simulink model "rmspec"  (Simulink 7.0)
settings: Solver=ode45  StartTime=0.0  StopTime=200  RelTol=1e-3
undefined symbols (not defined in the file): pfb_coeff_gen_calc
libraries: xbsIndex_r4 x3092, casper_library x230, xps_library x24
(part 1 of 33)
settings Model: Creator=dave  LastModifiedBy=dave

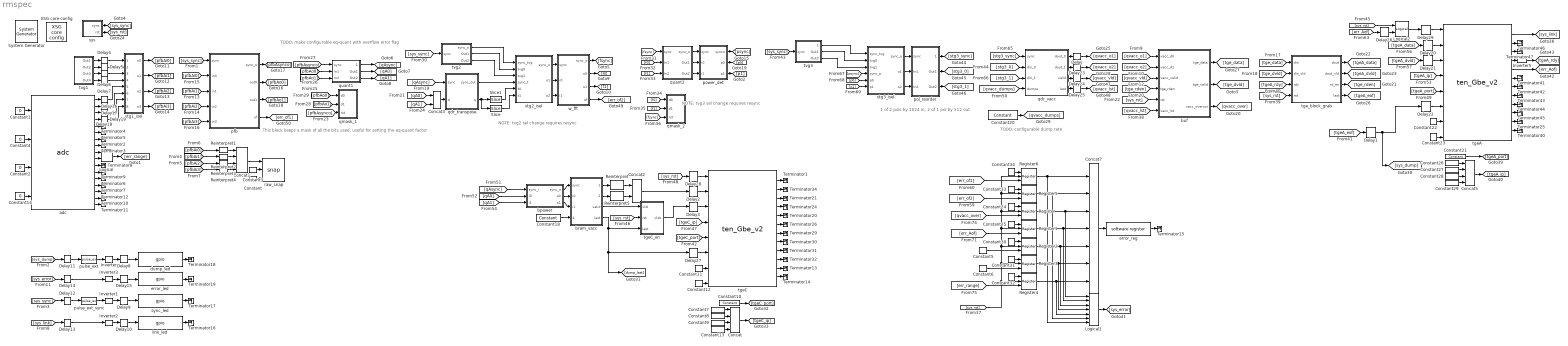
== system rmspec ==
  note: TODO: make configurable eq-quant with
      | overflow error flag
  note: This block keeps a mask of all the bits used,
      | useful for setting the eq-quant factor
  note: NOTE: tvg2 sel change
      | requires resync
  note: 1 of 2 pols by 1024 in,
      | 2 of 1 pol by 512 out
  note: NOTE: tvg3 sel change
      | requires resync
  note: TODO: configurable dump rate
  " System Generator" : xbsIndex_r4/ System Generator  Tag=genX  SystemSampleTime=-1  xilinxfamily=virtex5  part=xc5vsx95t  speed=-1  package=ff1136  synthesis_tool=XST  clock_wrapper=Clock Enables  directory=./rmspec/sysgen  testbench=off  simulink_period=1  sysclk_period=5  dcm_input_clock_period=100  incr_netlist=off  trim_vbits=Everywhere in SubSystem  dbl_ovrd=According to Block Masks  core_generation=According to Block Masks  run_coregen=off  deprecated_control=off  eval_field=0  block_type=sysgen
      settings: block_version=10.1.3
  Concat : xbsIndex_r4/Concat  num_inputs=4  dbl_ovrd=off  block_type=concat
      settings: block_version=10.1.3
  Concat1 : xbsIndex_r4/Concat  num_inputs=4  dbl_ovrd=off  block_type=concat
      settings: block_version=10.1.3
  Concat2 : xbsIndex_r4/Concat  num_inputs=2  dbl_ovrd=off  block_type=concat
      settings: block_version=10.1.3
  Concat3 : xbsIndex_r4/Concat  num_inputs=2  dbl_ovrd=off  block_type=concat
      settings: block_version=10.1.3
  Concat5 : xbsIndex_r4/Concat  num_inputs=4  dbl_ovrd=off  block_type=concat
      settings: block_version=10.1.3
  Concat7 : xbsIndex_r4/Concat  num_inputs=7  dbl_ovrd=off  block_type=concat
      settings: block_version=10.1.3
  Constant : xbsIndex_r4/Constant  arith_type=Boolean  const=1  n_bits=16  bin_pt=14  explicit_period=on  period=1  equ=P=C  opselect=C  inp2=PCIN>>17  opr=+  inp1=P  carry=CIN  dbl_ovrd=off  block_type=constant
  Constant{1..2,4,14} (4 alike) : Constant  Value=0  OutDataType=sfix(16)  OutScaling=2^0
  Constant10 : xbsIndex_r4/Constant  arith_type=Unsigned  const=10002  n_bits=16  bin_pt=0  explicit_period=off  period=1  equ=P=C  opselect=C  inp2=PCIN>>17  opr=+  inp1=P  carry=CIN  dbl_ovrd=off  block_type=constant
  Constant{11..12,22..25,30..34} (11 alike) : xbsIndex_r4/Constant  arith_type=Boolean  const=1  n_bits=16  bin_pt=14  explicit_period=off  period=1  equ=P=C  opselect=C  inp2=PCIN>>17  opr=+  inp1=P  carry=CIN  dbl_ovrd=off  block_type=constant
  Constant13 : xbsIndex_r4/Constant  arith_type=Unsigned  const=2  n_bits=8  bin_pt=0  explicit_period=off  period=1  equ=P=C  opselect=C  inp2=PCIN>>17  opr=+  inp1=P  carry=CIN  dbl_ovrd=off  block_type=constant
  Constant18 : xbsIndex_r4/Constant  arith_type=Unsigned  const=2^23 - 2  n_bits=32  bin_pt=0  explicit_period=off  period=1  equ=P=C  opselect=C  inp2=PCIN>>17  opr=+  inp1=P  carry=CIN  dbl_ovrd=off  block_type=constant
  Constant20 : xbsIndex_r4/Constant  arith_type=Unsigned  const=(2^10)*(2^(10-1))*(2^9) - 2  n_bits=32  bin_pt=0  explicit_period=on  period=1  equ=P=C  opselect=C  inp2=PCIN>>17  opr=+  inp1=P  carry=CIN  dbl_ovrd=off  block_type=constant
  Constant21 : xbsIndex_r4/Constant  arith_type=Unsigned  const=10000  n_bits=16  bin_pt=0  explicit_period=off  period=1  equ=P=C  opselect=C  inp2=PCIN>>17  opr=+  inp1=P  carry=CIN  dbl_ovrd=off  block_type=constant
  Constant26 : xbsIndex_r4/Constant  arith_type=Unsigned  const=192  n_bits=8  bin_pt=0  explicit_period=off  period=1  equ=P=C  opselect=C  inp2=PCIN>>17  opr=+  inp1=P  carry=CIN  dbl_ovrd=off  block_type=constant
  Constant27 : xbsIndex_r4/Constant  arith_type=Unsigned  const=168  n_bits=8  bin_pt=0  explicit_period=off  period=1  equ=P=C  opselect=C  inp2=PCIN>>17  opr=+  inp1=P  carry=CIN  dbl_ovrd=off  block_type=constant
  Constant28 : xbsIndex_r4/Constant  arith_type=Unsigned  const=5  n_bits=8  bin_pt=0  explicit_period=off  period=1  equ=P=C  opselect=C  inp2=PCIN>>17  opr=+  inp1=P  carry=CIN  dbl_ovrd=off  block_type=constant
  Constant29 : xbsIndex_r4/Constant  arith_type=Unsigned  const=2  n_bits=8  bin_pt=0  explicit_period=off  period=1  equ=P=C  opselect=C  inp2=PCIN>>17  opr=+  inp1=P  carry=CIN  dbl_ovrd=off  block_type=constant
  Constant3 : xbsIndex_r4/Constant  arith_type=Boolean  const=0  n_bits=16  bin_pt=14  explicit_period=on  period=1  equ=P=C  opselect=C  inp2=PCIN>>17  opr=+  inp1=P  carry=CIN  dbl_ovrd=off  block_type=constant
  Constant5 : xbsIndex_r4/Constant  arith_type=Boolean  const=0  n_bits=16  bin_pt=14  explicit_period=on  period=1  equ=P=C  opselect=C  inp2=PCIN>>17  opr=+  inp1=P  carry=CIN  dbl_ovrd=off  block_type=constant
  Constant6 : xbsIndex_r4/Constant  arith_type=Boolean  const=0  n_bits=16  bin_pt=14  explicit_period=on  period=1  equ=P=C  opselect=C  inp2=PCIN>>17  opr=+  inp1=P  carry=CIN  dbl_ovrd=off  block_type=constant
  Constant7 : xbsIndex_r4/Constant  arith_type=Unsigned  const=192  n_bits=8  bin_pt=0  explicit_period=off  period=1  equ=P=C  opselect=C  inp2=PCIN>>17  opr=+  inp1=P  carry=CIN  dbl_ovrd=off  block_type=constant
  Constant8 : xbsIndex_r4/Constant  arith_type=Unsigned  const=168  n_bits=8  bin_pt=0  explicit_period=off  period=1  equ=P=C  opselect=C  inp2=PCIN>>17  opr=+  inp1=P  carry=CIN  dbl_ovrd=off  block_type=constant
  Constant9 : xbsIndex_r4/Constant  arith_type=Unsigned  const=5  n_bits=8  bin_pt=0  explicit_period=off  period=1  equ=P=C  opselect=C  inp2=PCIN>>17  opr=+  inp1=P  carry=CIN  dbl_ovrd=off  block_type=constant
  Delay{,1,4..19,22..26} (23 alike) : xbsIndex_r4/Delay  en=off  latency=1  dbl_ovrd=off  reg_retiming=off  block_type=delay
  Delay{2..3,20..21,27..29} (7 alike) : xbsIndex_r4/Delay  en=off  latency=2  dbl_ovrd=off  reg_retiming=off  block_type=delay
  Inverter{,1..3,5} (5 alike) : xbsIndex_r4/Inverter  en=off  latency=0  dbl_ovrd=off  block_type=inv
  Logical : xbsIndex_r4/Logical  logical_function=OR  inputs=2  en=off  latency=0  precision=Full  arith_type=Unsigned  n_bits=16  bin_pt=0  align_bp=on  dbl_ovrd=off  block_type=logical
  Logical1 : xbsIndex_r4/Logical  logical_function=OR  inputs=7  en=off  latency=1  precision=Full  arith_type=Unsigned  n_bits=16  bin_pt=0  align_bp=on  dbl_ovrd=off  block_type=logical
  Logical2 : xbsIndex_r4/Logical  logical_function=OR  inputs=2  en=off  latency=0  precision=Full  arith_type=Unsigned  n_bits=16  bin_pt=0  align_bp=on  dbl_ovrd=off  block_type=logical
  Register{,1..6} (7 alike) : xbsIndex_r4/Register  init=0  rst=on  en=on  dbl_ovrd=off  block_type=register
  Reinterpret{,1..5} (6 alike) : xbsIndex_r4/Reinterpret  force_arith_type=on  arith_type=Unsigned  force_bin_pt=on  bin_pt=0  block_type=reinterpret
      settings: infoedit="Changes signal type without altering the binary representation.   You can changed the signal between signed and unsigned, and relocate the binary point.<P><P>Hardware notes: In hardware this block costs nothing.<P><P>Example:  Suppose the input is 6 bits wide, signed, with 2 fractional bits, and the output is forced to unsigned with 0 fractional bits.  Then an input of -2.0 (1110.00 in binary 2's complement) becomes an output of 56 (111000 in binary)."  block_version=10.1.3
  Slice : xbsIndex_r4/Slice  nbits=18  boolean_output=off  mode=Lower Bit Location + Width  bit1=0  base1=LSB of Input  bit0=0  base0=LSB of Input  dbl_ovrd=off  block_type=slice
      settings: infoedit="Extracts a given range of bits from each input sample and presents it at the output.  The output type is ordinarily unsigned with binary point at zero, but can be Boolean when the slice is one bit wide.<P><P>Hardware notes: In hardware this block costs nothing."  block_version=10.1.3
  Slice1 : xbsIndex_r4/Slice  nbits=18  boolean_output=off  mode=Lower Bit Location + Width  bit1=0  base1=LSB of Input  bit0=18  base0=LSB of Input  dbl_ovrd=off  block_type=slice
      settings: infoedit="Extracts a given range of bits from each input sample and presents it at the output.  The output type is ordinarily unsigned with binary point at zero, but can be Boolean when the slice is one bit wide.<P><P>Hardware notes: In hardware this block costs nothing."  block_version=10.1.3
  Terminator{1..21,24..26,29..32,34,40..47} (37 alike) : Terminator
  XSG core config : xps_library/XSG core config  Tag=xps:xsg  SystemSampleTime=-1  hw_sys=ROACH:sx95t  ibob_linux=off  clk_src=adc0_clk  iBOB_clk_src=sys_clk  BEE2_ctrl_clk_src=sys_clk  BEE2_usr_clk_src=sys_clk  ROACH_clk_src=adc0_clk  CORR_clk_src=sys_clk  gpio_clk_io_group=iBOB:sma  gpio_clk_bit_index=0  clk_rate=200  sample_period=1  synthesis_tool=XST  mpc_type=powerpc440_ext
  adc : xps_library/adc  Tag=xps:adc  SystemSampleTime=-1  adc_brd=adc0  adc_clk_rate=800  adc_interleave=off  sample_period=1
  bpower : Subsystem  mask{bits=9}
  bram_vacc : Subsystem  mask{n_chans=512}
      mask prompts: n_chans "Number of Channels"
  buf : Subsystem  mask{fftsize=10, nochan=10}
      mask prompts: fftsize "fftsize (2^n)"; nochan "nochan (2^n)"
  dump_led : xps_library/gpio  Tag=xps:gpio  SystemSampleTime=-1  io_group=ROACH:led  io_dir=out  arith_type=Boolean  bitwidth=1  bin_pt=0  bit_index=0  sample_period=1  use_single_ended=off  use_ddr=off  reg_iob=on  reg_clk_phase=0  termination=None
      link override convert: arith_type=Boolean  n_bits=1  bin_pt=0
  error_led : xps_library/gpio  Tag=xps:gpio  SystemSampleTime=-1  io_group=ROACH:led  io_dir=out  arith_type=Boolean  bitwidth=1  bin_pt=0  bit_index=1  sample_period=1  use_single_ended=off  use_ddr=off  reg_iob=on  reg_clk_phase=0  termination=None
      link override convert: arith_type=Boolean  n_bits=1  bin_pt=0
  error_reg : xps_library/software register  Tag=xps:sw_reg  SystemSampleTime=-1  io_dir=To Processor  arith_type=Unsigned  bitwidth=32  bin_pt=0  sample_period=1  gw_name=rmspec_error_reg_user_data_in
      link override convert: arith_type=Unsigned  n_bits=32  bin_pt=0
  link_led : xps_library/gpio  Tag=xps:gpio  SystemSampleTime=-1  io_group=ROACH:led  io_dir=out  arith_type=Boolean  bitwidth=1  bin_pt=0  bit_index=3  sample_period=1  use_single_ended=off  use_ddr=off  reg_iob=on  reg_clk_phase=0  termination=None
      link override convert: arith_type=Boolean  n_bits=1  bin_pt=0
  pfb : Subsystem
  pol_reorder : Subsystem
  power_det : Subsystem
  pulse_ext : casper_library/Misc/pulse_ext  SystemSampleTime=-1  pulse_len=2^25
  pulse_ext_sync : casper_library/Misc/pulse_ext  SystemSampleTime=-1  pulse_len=2^20
  qdr_transpose : Subsystem  AncestorBlock=casper_library/Reorder/qdr_transpose  mask{idepth=9, odepth=10, which_qdr=qdr0}
      link override reorder: map=[0 1 2 3]  n_inputs=2
      mask prompts: idepth "Input blocksize (2^n)"; odepth "Output blocksize (2^n)"; which_qdr "QDR Chip"
      mask init:
      | new_map = tostring([[0:2^odepth-1]*2 [0:2^odepth-1]*2 + 1]);
      | set_param([gcb, '/reorder'], 'map', new_map);
      | set_param([gcb, '/qdr'], 'which_qdr', which_qdr);
      mask StyleString: edit,edit,popup(qdr0|qdr1)
  qdr_vacc : Subsystem  mask{n_chans=(2^10)*(2^(10-1)), which_qdr=1, add_lat=3}
      mask prompts: n_chans "Vector Length"; which_qdr "QDR Chip"; add_lat "add_latency"
      mask init:
      | set_param([gcb, '/qdr_delay'], 'which_qdr', sprintf('%d',which_qdr));
  qmask_1 : Subsystem
  qmask_2 : Subsystem
  quant1 : Subsystem  mask{fact=0, bits=9}
      mask prompts: fact "fact (2^n)"; bits "quant bits"
  quant2 : Subsystem  mask{fact=0, bits=18}
      mask prompts: fact "fact (2^n)"; bits "quant bits"
  raw_snap : casper_library/Scopes/snap  SystemSampleTime=-1  nsamples=11
      link override addr/convert: arith_type=Unsigned  n_bits=32  bin_pt=0
      link override bram/convert_din: arith_type=Unsigned
      link override bram/mem/sim_data_in: arith_type=Unsigned
      link override bram/pfb1_tv_raw_snap_bram_data_out: arith_type=Unsigned
      link override bram/rmspec_raw_snap_bram_data_out: arith_type=Unsigned
      link override bram/roach_mspec_raw_snap_bram_data_out: arith_type=Unsigned
      link override bram/stg1_raw_snap_bram_data_out: arith_type=Unsigned
      link override ctrl/pfb1_tv_raw_snap_ctrl_user_data_out: arith_type=Unsigned  n_bits=32  bin_pt=0  period=1
      link override ctrl/rmspec_raw_snap_ctrl_user_data_out: arith_type=Unsigned  n_bits=32  bin_pt=0  period=1
      link override ctrl/roach_mspec_raw_snap_ctrl_user_data_out: arith_type=Unsigned  n_bits=32  bin_pt=0  period=1
      link override ctrl/stg1_raw_snap_ctrl_user_data_out: arith_type=Unsigned  n_bits=32  bin_pt=0  period=1
  stg1_isel : Subsystem
  stg2_isel : Subsystem
  stg3_isel : Subsystem
  sync_led : xps_library/gpio  Tag=xps:gpio  SystemSampleTime=-1  io_group=ROACH:led  io_dir=out  arith_type=Boolean  bitwidth=1  bin_pt=0  bit_index=2  sample_period=1  use_single_ended=off  use_ddr=off  reg_iob=on  reg_clk_phase=0  termination=None
      link override convert: arith_type=Boolean  n_bits=1  bin_pt=0
  sys : Subsystem
  tgeA : xps_library/ten_Gbe_v2  Tag=xps:tengbe_v2  SystemSampleTime=-1  port=0  rx_dist_ram=on  show_param=on  pre_emph=3  swing=800  fab_en=on  fab_mac=hex2dec('123456780000')  fab_ip=192*(2^24) + 168*(2^16) + 5*(2^8) + 20*(2^0)  fab_udp=10000  fab_gate=1  cpu_rx_en=off  cpu_tx_en=off
  tgeC : xps_library/ten_Gbe_v2  Tag=xps:tengbe_v2  SystemSampleTime=-1  port=2  rx_dist_ram=on  show_param=on  pre_emph=3  swing=800  fab_en=on  fab_mac=hex2dec('123456780002')  fab_ip=192*(2^24) + 168*(2^16) + 5*(2^8) + 20*(2^0)  fab_udp=10002  fab_gate=1  cpu_rx_en=off  cpu_tx_en=off
  tgeC_en : Subsystem
  tge_block_grab : Subsystem
  tvg1 : Subsystem  mask{lev=0.1}
  tvg2 : Subsystem
  tvg3 : Subsystem  mask{fftsize=10, nochan=10, vaccwidth=18, dumps=9}
      mask prompts: fftsize "fftsize (2^n)"; nochan "nochan (2^n)"; dumps "dumps (2^n)"
  w_fft : Subsystem
  wires:
  [pfbAi0] -> Reinterpret1/1
  [pfbAi1] -> Reinterpret2/1
  [pfbAi2] -> Reinterpret3/1
  [pfbAi3] -> Reinterpret4/1
  Concat1/1 -> raw_snap/1
  Constant/1 -> raw_snap/3
  Constant3/1 -> raw_snap/2
  Reinterpret1/1 -> Concat1/1
  Reinterpret2/1 -> Concat1/2
  Reinterpret3/1 -> Concat1/3
  Reinterpret4/1 -> Concat1/4
  [pfbAo0] -> quant1/2(In1)
  [pfbAo1] -> quant1/3(In2)
  [pfbAsynco] -> quant1/1(sync)
  [pfbAi0] -> pfb/2(in0)
  [pfbAi1] -> pfb/3(in1)
  [pfbAi2] -> pfb/4(in2)
  [pfbAi3] -> pfb/5(in3)
  pfb/1(sync_o) -> [pfbAsynco]
  pfb/2(out0) -> [pfbAo0]
  pfb/3(out1) -> [pfbAo1]
  [sys_sync] -> pfb/1(sync)
  pulse_ext/1 -> Inverter/1
  [sys_dump] -> Delay11/1
  [sys_sync] -> Delay12/1
  [sys_link] -> Delay13/1
  tvg1/1(Out1) -> Delay4/1
  tvg1/2(Out2) -> Delay5/1
  tvg1/3(Out3) -> Delay6/1
  tvg1/4(Out4) -> Delay7/1
  pfb/4(of) -> [err_of1]
  Delay8/1 -> dump_led/1
  Delay9/1 -> sync_led/1
  Delay10/1 -> link_led/1
  Delay11/1 -> pulse_ext/1
  Delay12/1 -> pulse_ext_sync/1
  Delay13/1 -> Inverter2/1
  Inverter/1 -> Delay8/1
  Inverter1/1 -> Delay9/1
  Inverter2/1 -> Delay10/1
  quant1/1(sync_o) -> [qAsync]
  quant1/2(Out1) -> [qA0]
  quant1/3(Out2) -> [qA1]
  Constant1/1 -> adc/1
  Constant2/1 -> adc/3
  Constant4/1 -> adc/2
  Constant14/1 -> adc/4
  adc/1 -> Delay16/1
  adc/2 -> Delay17/1
  adc/3 -> Delay18/1
  adc/4 -> Delay19/1
  adc/5 -> Terminator4/1
  adc/6 -> Terminator5/1
  adc/7 -> Terminator2/1
  adc/8 -> Terminator3/1
  sys/1(sync) -> [sys_sync]
  sys/2(rst) -> [sys_rst]
  adc/9 -> Logical/1
  adc/10 -> Logical/2
  stg1_isel/1(o0) -> [pfbAi0]
  stg1_isel/2(o1) -> [pfbAi1]
  stg1_isel/3(o2) -> [pfbAi2]
  stg1_isel/4(o3) -> [pfbAi3]
  Logical/1 -> [err_range]
  adc/11 -> Terminator8/1
  adc/12 -> Terminator9/1
  adc/13 -> Terminator6/1
  adc/14 -> Terminator7/1
  adc/15 -> Terminator12/1
  adc/16 -> Terminator10/1
  adc/17 -> Terminator11/1
  Delay16/1 -> stg1_isel/5(adc0)
  Delay17/1 -> stg1_isel/6(adc1)
  Delay18/1 -> stg1_isel/7(adc2)
  Delay19/1 -> stg1_isel/8(adc3)
  dump_led/1 -> Terminator18/1
  sync_led/1 -> Terminator17/1
  link_led/1 -> Terminator16/1
  [sys_error] -> Delay14/1
  Delay15/1 -> error_led/1
  Delay14/1 -> Inverter3/1
  Inverter3/1 -> Delay15/1
  error_led/1 -> Terminator19/1
  [pfbAo0] -> qmask_1/1(d0)
  [pfbAo1] -> qmask_1/2(d1)
  [pfbAsynco] -> qmask_1/3(rst)
  Delay4/1 -> stg1_isel/1(tvg0)
  Delay5/1 -> stg1_isel/2(tvg1)
  Delay6/1 -> stg1_isel/3(tvg2)
  Delay7/1 -> stg1_isel/4(tvg3)
  pulse_ext_sync/1 -> Inverter1/1
  [qA0] -> Concat3/1
  [qA1] -> Concat3/2
  [qAsync] -> qdr_transpose/1(sync)
  Concat3/1 -> qdr_transpose/2(d)
  qdr_transpose/2(q) -> Slice1/1, Slice/1
  [sys_sync] -> tvg2/1(sync)
  tvg2/1(sync_o) -> stg2_isel/1(sync_tvg)
  tvg2/2(Out1) -> stg2_isel/2(tvg0)
  tvg2/3(Out2) -> stg2_isel/3(tvg1)
  qdr_transpose/1(sync_out) -> stg2_isel/4(sync_t)
  Slice1/1 -> stg2_isel/5(t0)
  Slice/1 -> stg2_isel/6(t1)
  stg2_isel/1(sync_o) -> w_fft/1(sync)
  stg2_isel/2(o1) -> w_fft/2(i0)
  stg2_isel/3(o2) -> w_fft/3(i1)
  w_fft/1(sync_o) -> [fsync]
  w_fft/2(o0) -> [f0]
  w_fft/3(o1) -> [f1]
  [fsync] -> quant2/1(sync)
  [f0] -> quant2/2(In1)
  [f1] -> quant2/3(In2)
  [f0] -> qmask_2/1(d0)
  [f1] -> qmask_2/2(d1)
  [fsync] -> qmask_2/3(rst)
  power_det/1(synco) -> [psync]
  power_det/2(p0) -> [p0]
  power_det/3(p1) -> [p1]
  [qvacc_dumps] -> qdr_vacc/4(dumps)
  [sys_sync] -> tvg3/1(sync)
  tgeA/1 -> [sys_link]
  tgeA/2 -> Terminator46/1
  [tgeA_ip] -> tgeA/4
  [tgeA_port] -> tgeA/5
  Constant26/1 -> Concat5/1
  Constant27/1 -> Concat5/2
  Constant28/1 -> Concat5/3
  Constant29/1 -> Concat5/4
  Concat5/1 -> [tgeA_ip]
  Constant21/1 -> [tgeA_port]
  tgeA/4 -> Inverter5/1
  tgeA/6 -> Terminator41/1
  tgeA/7 -> Terminator42/1
  tgeA/8 -> Terminator43/1
  tgeA/9 -> Terminator44/1
  tgeA/10 -> Terminator45/1
  tgeA/11 -> Terminator25/1
  tgeA/12 -> Terminator40/1
  Constant22/1 -> tgeA/7
  Constant23/1 -> tgeA/8
  Delay20/1 -> tgeA/2
  Delay21/1 -> tgeA/3
  Delay22/1 -> tgeA/6
  tgeA/5 -> [err_Aof]
  [err_Aof] -> Delay26/1
  Inverter5/1 -> [tgeA_rdy]
  [stg3_sync] -> qdr_vacc/1(sync)
  [stg3_0] -> qdr_vacc/2(din_0)
  [stg3_1] -> qdr_vacc/3(din_1)
  qdr_vacc/1(dout_0) -> Delay/1
  qdr_vacc/2(dout_1) -> Delay23/1
  qdr_vacc/3(valid) -> Delay24/1
  Constant20/1 -> [qvacc_dumps]
  [tgeA_data] -> Delay20/1
  [tgeA_dvld] -> Delay21/1
  Constant24/1 -> Register/1
  Constant25/1 -> Register1/1
  Register/1 -> Concat7/3, Logical1/1
  Register1/1 -> Concat7/4, Logical1/2
  Logical1/1 -> [sys_error]
  error_reg/1 -> Terminator15/1
  Delay/1 -> [qvacc_o1]
  Delay23/1 -> [qvacc_o2]
  pol_reorder/1(sync_o) -> [stg3_sync]
  pol_reorder/2(Out1) -> [stg3_0]
  pol_reorder/3(Out2) -> [stg3_1]
  Delay24/1 -> [qvacc_vld]
  Delay25/1 -> [qvacc_lst]
  qdr_vacc/4(last) -> Delay25/1
  [sys_rst] -> Logical2/1
  Delay26/1 -> Logical2/2
  Logical2/1 -> Delay29/1
  [psync] -> stg3_isel/4(sync_p)
  [p0] -> stg3_isel/5(p0)
  tvg3/1(sync_o) -> stg3_isel/1(sync_tvg)
  tvg3/2(Out1) -> stg3_isel/2(tvg0)
  tvg3/3(Out2) -> stg3_isel/3(tvg1)
  [p1] -> stg3_isel/6(p1)
  stg3_isel/1(sync_o) -> pol_reorder/1(sync)
  stg3_isel/2(o1) -> pol_reorder/2(In1)
  stg3_isel/3(o2) -> pol_reorder/3(In2)
  tgeA/3 -> Terminator47/1
  Constant30/1 -> Register2/1
  Constant31/1 -> Register3/1
  Register2/1 -> Concat7/5, Logical1/3
  Register3/1 -> Concat7/6, Logical1/4
  Constant32/1 -> Register4/1
  Register4/1 -> Concat7/7, Logical1/5
  Delay29/1 -> tgeA/1
  w_fft/4(of) -> [err_of2]
  Constant33/1 -> Register5/1
  Constant34/1 -> Register6/1
  Concat7/1 -> error_reg/1
  Register6/1 -> Concat7/1, Logical1/7
  Register5/1 -> Concat7/2, Logical1/6
  [sys_rst] -> Register6/2, Register5/2, Register/2, Register1/2, Register2/2, Register3/2, Register4/2
  [err_of1] -> Register6/3
  [err_of2] -> Register5/3
  [qvacc_over] -> Register/3
  [err_Aof] -> Register1/3
  Constant6/1 -> Register3/3
  [err_range] -> Register4/3
  Constant5/1 -> Register2/3
  [tgeA_rdy] -> tge_block_grab/3(rdy)
  buf/1(tge_data) -> [tge_data]
  buf/2(tge_valid) -> [tge_dvld]
  buf/3(vacc_overrun) -> [qvacc_over]
  [tge_data] -> tge_block_grab/1(din)
  [tge_dvld] -> tge_block_grab/2(din_vld)
  tge_block_grab/3(rd_en) -> [tge_rden]
  tge_block_grab/1(dout) -> [tgeA_data]
  tge_block_grab/2(dout_vld) -> [tgeA_dvld]
  tge_block_grab/4(last) -> [tgeA_eof]
  [qvacc_o1] -> buf/1(vacc_d0)
  [qvacc_o2] -> buf/2(vacc_d1)
  [qvacc_vld] -> buf/3(vacc_valid)
  [tge_rden] -> buf/4(tge_rden)
  [sys_rst] -> buf/5(rst)
  [qvacc_lst] -> buf/6(vacc_lst)
  [sys_rst] -> tge_block_grab/4(rst)
  [tgeA_eof] -> Delay1/1
  Delay1/1 -> Delay22/1, [sys_dump]
  Constant18/1 -> bram_vacc/4(dumps)
  tgeC/1 -> Terminator1/1
  tgeC/2 -> Terminator34/1
  tgeC/3 -> Terminator21/1
  [tgeC_ip] -> tgeC/4
  [tgeC_port] -> tgeC/5
  Constant7/1 -> Concat/1
  Constant8/1 -> Concat/2
  Constant9/1 -> Concat/3
  Constant13/1 -> Concat/4
  Concat/1 -> [tgeC_ip]
  Constant10/1 -> [tgeC_port]
  tgeC/4 -> Terminator24/1
  tgeC/6 -> Terminator26/1
  tgeC/7 -> Terminator29/1
  tgeC/8 -> Terminator30/1
  tgeC/9 -> Terminator31/1
  tgeC/10 -> Terminator32/1
  tgeC/11 -> Terminator13/1
  tgeC/12 -> Terminator14/1
  Constant11/1 -> tgeC/7
  Constant12/1 -> tgeC/8
  Delay2/1 -> tgeC/2
  Delay3/1 -> tgeC/3
  Delay27/1 -> tgeC/6
  tgeC/5 -> Terminator20/1
  bpower/1(sync_o) -> bram_vacc/1(sync)
  bpower/2(o0) -> bram_vacc/2(i0)
  bpower/3(o1) -> bram_vacc/3(i1)
  [sys_rst] -> Delay28/1
  bram_vacc/1(dout_0) -> Reinterpret/1
  bram_vacc/2(dout_1) -> Reinterpret5/1
  [sys_rst] -> tgeC_en/2(rst)
  bram_vacc/3(valid) -> tgeC_en/1(vldi)
  bram_vacc/4(last) -> tgeC_en/3(last), Delay27/1, [dump_last]
  Concat2/1 -> Delay2/1
  tgeC_en/1(vldo) -> Delay3/1
  Reinterpret/1 -> Concat2/1
  Reinterpret5/1 -> Concat2/2
  Delay28/1 -> tgeC/1
  [qAsync] -> bpower/1(sync_i)
  [qA0] -> bpower/2(i0)
  [qA1] -> bpower/3(i1)
  quant2/1(sync_o) -> power_det/1(sync)
  quant2/2(Out1) -> power_det/2(i0)
  quant2/3(Out2) -> power_det/3(i1)

== system rmspec/bpower ==
  sync_i : Inport
  i0 : Inport  Port=2
  i1 : Inport  Port=3
  Delay : xbsIndex_r4/Delay  en=off  latency=3  dbl_ovrd=off  reg_retiming=off  block_type=delay
  Scope : Scope  NumInputPorts=3
      settings: YMin=-5~-5~-5  YMax=5~5~5
  power0 : casper_library/Misc/power  SystemSampleTime=-1  BitWidth=bits  add_latency=1  mult_latency=2
  power1 : casper_library/Misc/power  SystemSampleTime=-1  BitWidth=bits  add_latency=1  mult_latency=2
      link override power_adder: mode=Addition  use_carryin=off  use_carryout=off  en=off  latency=add_latency  precision=User Defined  arith_type=Unsigned  n_bits=BitWidth * 2  bin_pt=BitWidth * 2 - 1  quantization=Truncate  overflow=Saturate  dbl_ovrd=off  use_behavioral_HDL=on  pipelined=off  use_rpm=on  hw_selection=Fabric
      link override power_adder: xl_area=[0, 0, 0, 0, 0, 0, 0]
  sync_o : Outport
  o0 : Outport  Port=2
  o1 : Outport  Port=3
  wires:
  sync_i/1 -> Delay/1
  Delay/1 -> sync_o/1, Scope/1
  i0/1 -> power0/1
  i1/1 -> power1/1
  power0/1 -> o0/1, Scope/2
  power1/1 -> o1/1, Scope/3

== system rmspec/bram_vacc ==
  sync : Inport
  i0 : Inport  Port=2
  i1 : Inport  Port=3
  dumps : Inport  Port=4
  Constant2 : xbsIndex_r4/Constant  arith_type=Unsigned  const=0  n_bits=32  bin_pt=0  explicit_period=on  period=1  equ=P=C  opselect=C  inp2=PCIN>>17  opr=+  inp1=P  carry=CIN  dbl_ovrd=off  block_type=constant
  Delay1 : xbsIndex_r4/Delay  en=off  latency=1  dbl_ovrd=off  reg_retiming=off  block_type=delay
  Delay2 : xbsIndex_r4/Delay  en=off  latency=1  dbl_ovrd=off  reg_retiming=off  block_type=delay
  Logical : xbsIndex_r4/Logical  logical_function=OR  inputs=2  en=off  latency=0  precision=Full  arith_type=Unsigned  n_bits=16  bin_pt=0  align_bp=on  dbl_ovrd=off  block_type=logical
  Relational : xbsIndex_r4/Relational  mode=a=b  en=off  latency=1  dbl_ovrd=off  block_type=relational
      settings: block_version=10.1.3
  Relational2 : xbsIndex_r4/Relational  mode=a=b  en=off  latency=1  dbl_ovrd=off  block_type=relational
      settings: block_version=10.1.3
  Terminator2 : Terminator
  channel_counter : xbsIndex_r4/Counter  cnt_type=Free Running  cnt_to=Inf  operation=Up  start_count=0  cnt_by_val=1  arith_type=Unsigned  n_bits=32  bin_pt=0  load_pin=off  rst=on  en=off  explicit_period=on  period=1  dbl_ovrd=off  use_behavioral_HDL=off  use_rpm=off  implementation=Fabric  block_type=counter
  posedge1 : casper_library/Misc/posedge  Tag=Rising Edge Detector  SystemSampleTime=-1
  posedge2 : casper_library/Misc/posedge  Tag=Rising Edge Detector  SystemSampleTime=-1
  simple_bram_vacc : Subsystem  mask(simple_vacc){n_chans=512, n_bits=32, bin_pos=18}
      mask prompts: n_chans "Vector Length"; n_bits "Number of output bits"; bin_pos "Binary point (output)"
      mask help: This simple vector accumulator is based on a shift register. It outputs its previous accumulated vector after a new_acc pulse is received.
      mask init:
      | chan_bits=ceil(log2(n_chans));
  simple_bram_vacc1 : Subsystem  mask(simple_vacc){n_chans=512, n_bits=32, bin_pos=18}
      mask prompts: n_chans "Vector Length"; n_bits "Number of output bits"; bin_pos "Binary point (output)"
      mask help: This simple vector accumulator is based on a shift register. It outputs its previous accumulated vector after a new_acc pulse is received.
      mask init:
      | chan_bits=ceil(log2(n_chans));
  sync_delay : casper_library/Delays/sync_delay  SystemSampleTime=-1  DelayLen=n_chans -1
  dout_0 : Outport
  dout_1 : Outport  Port=2
  valid : Outport  Port=3
  last : Outport  Port=4
  wires:
  sync/1 -> posedge1/1
  channel_counter/1 -> Relational/2, Relational2/1
  simple_bram_vacc1/1(dout) -> dout_1/1
  Logical/1 -> channel_counter/1
  Relational/1 -> Logical/1
  Constant2/1 -> Relational2/2
  Relational2/1 -> simple_bram_vacc/1(new_acc), simple_bram_vacc1/1(new_acc)
  posedge1/1 -> Logical/2
  dumps/1 -> Relational/1
  simple_bram_vacc1/2(valid) -> Terminator2/1
  simple_bram_vacc/1(dout) -> dout_0/1
  i0/1 -> Delay2/1
  i1/1 -> Delay1/1
  simple_bram_vacc/2(valid) -> valid/1, posedge2/1
  sync_delay/1 -> last/1
  Delay2/1 -> simple_bram_vacc/2(din)
  Delay1/1 -> simple_bram_vacc1/2(din)
  posedge2/1 -> sync_delay/1

== system rmspec/buf ==
  vacc_d0 : Inport
  vacc_d1 : Inport  Port=2
  vacc_valid : Inport  Port=3
  tge_rden : Inport  Port=4
  rst : Inport  Port=5
  vacc_lst : Inport  Port=6
  Constant : xbsIndex_r4/Constant  arith_type=Boolean  const=1  n_bits=16  bin_pt=14  explicit_period=off  period=1  equ=P=C  opselect=C  inp2=PCIN>>17  opr=+  inp1=P  carry=CIN  dbl_ovrd=off  block_type=constant
  Inverter : xbsIndex_r4/Inverter  en=off  latency=0  dbl_ovrd=off  block_type=inv
  Logical : xbsIndex_r4/Logical  logical_function=AND  inputs=2  en=off  latency=0  precision=Full  arith_type=Unsigned  n_bits=16  bin_pt=0  align_bp=on  dbl_ovrd=off  block_type=logical
  Logical1 : xbsIndex_r4/Logical  logical_function=AND  inputs=2  en=off  latency=0  precision=Full  arith_type=Unsigned  n_bits=16  bin_pt=0  align_bp=on  dbl_ovrd=off  block_type=logical
  Register : xbsIndex_r4/Register  init=0  rst=on  en=on  dbl_ovrd=off  block_type=register
  dram_buf : Subsystem  mask{block_size=fftsize+(nochan-1)-2}
      mask prompts: block_size "Block Size (2^n)"
  rd_collect : Subsystem
  wr_collect : Subsystem
  tge_data : Outport
  tge_valid : Outport  Port=2
  vacc_overrun : Outport  Port=3
  wires:
  vacc_d0/1 -> wr_collect/1(d0)
  vacc_d1/1 -> wr_collect/2(d1)
  rd_collect/2(dout) -> tge_data/1
  rd_collect/3(dout_vld) -> tge_valid/1
  wr_collect/1(dout) -> dram_buf/2(wr_data)
  wr_collect/2(dvld) -> dram_buf/3(wr_vld), [wr_vld]
  tge_rden/1 -> rd_collect/3(rd_en)
  Inverter/1 -> Logical/1
  Logical/1 -> vacc_overrun/1
  rd_collect/1(din_ack) -> [rd_ack]
  [rd_ack] -> dram_buf/1(rd_ack)
  dram_buf/3(wr_ack) -> [wr_ack]
  [wr_ack] -> Inverter/1
  [wr_vld] -> Logical/2
  dram_buf/1(rd_data) -> rd_collect/1(din)
  dram_buf/2(rd_vld) -> rd_collect/2(din_vld)
  rst/1 -> [rst]
  [rst] -> wr_collect/4(rst)
  [rst] -> dram_buf/4(rst)
  [rst] -> rd_collect/4(rst)
  vacc_lst/1 -> [lst]
  Constant/1 -> Register/1
  [rst] -> Register/2
  [lst] -> Register/3
  Register/1 -> [en]
  [en] -> Logical1/1
  Logical1/1 -> wr_collect/3(vld)
  vacc_valid/1 -> Logical1/2

== system rmspec/pfb ==
  sync : Inport
  in0 : Inport  Port=2
  in1 : Inport  Port=3
  in2 : Inport  Port=4
  in3 : Inport  Port=5
  Constant1 : xbsIndex_r4/Constant  arith_type=Unsigned  const=2047  n_bits=11  bin_pt=0  explicit_period=on  period=1  equ=P=C  opselect=C  inp2=PCIN>>17  opr=+  inp1=P  carry=CIN  dbl_ovrd=off  block_type=constant
  Delay1 : xbsIndex_r4/Delay  en=off  latency=1  dbl_ovrd=off  reg_retiming=off  block_type=delay
  Shift{4..7} (4 alike) : xbsIndex_r4/Shift  shift_dir=Right  shift_bits=1  en=off  latency=1  precision=Full  arith_type="Signed  (2's comp)"  n_bits=16  bin_pt=14  quantization=Truncate  overflow=Wrap  dbl_ovrd=off  block_type=shift
      settings: block_version=10.1.3
  fft_wideband_real1 : Subsystem  AncestorBlock=casper_library/FFTs/fft_wideband_real  mask(fft_wideband_real){FFTSize=11, input_bit_width=25, coeff_bit_width=18, n_inputs=2, quantization=Truncate, overflow=Wrap, add_latency=3, mult_latency=3, bram_latency=2, arch=Virtex5, opt_target=Logic, coeffs_bit_limit=8, delays_bit_limit=9, specify_mult=off, mult_spec=[2 2 2 2]}
      mask prompts: FFTSize "Size of FFT: (2^?)"; input_bit_width "Input/Output Bit Width"; coeff_bit_width "Coefficient Bit Width"; n_inputs "Number of Simultaneous Inputs: (2^?)"; quantization "Quantization Behavior"; overflow "Overflow Behavior"; add_latency "Add Latency"; mult_latency "Mult Latency"; bram_latency "BRAM Latency"; arch "Architecture"; opt_target "Optimisation Target"; coeffs_bit_limit "Number bits above which to store stage's coefficients in BRAM (2^? bits)"; delays_bit_limit "Number bits above which to store stage's delays in BRAM (2^? bits)"; specify_mult "Specify multiplier use (behavioral HDL if not specified)"; mult_spec "Multiplier specification (0=core, 1=embedded, 2=behavioural) (left=1st stage)"
      mask init:
      | fft_wideband_real_init(gcb,...
      |     'FFTSize', FFTSize,...
      |     'input_bit_width', input_bit_width,...
      |     'coeff_bit_width', coeff_bit_width,...
      |     'n_inputs', n_inputs,...
      |     'quantization', quantization,...
      |     'overflow', overflow,...
      |     'add_latency', add_latency,...
      |     'mult_latency', mult_latency,...
      |     'bram_latency', bram_latency,...
      |     'arch', arch, ...
      |     'opt_target', opt_target, ...
      |     'coeffs_bit_limit', coeffs_bit_limit, ...
      |     'delays_bit_limit', delays_bit_limit, ...    
      |     'specify_mult', specify_mult,...
      |     'mult_spec', mult_spec);
      settings: AttributesFormatString=FFTSize=11
      mask Help: eval('xlWeb([getenv(''MLIB_ROOT''), ''\doc\htmlblocks\sp_fft_wideband_real\sp_fft_wideband_real.html''])')
      mask StyleString: edit,edit,edit,edit,popup(Truncate|Round  (unbiased: +/- Inf)|Round  (unbiased: Even Values)),popup(Wrap|Saturate|Error),edit,edit,edit,popup(Virtex2Pro|Virtex5),popup(Logic|Multipliers),edit,edit,checkbox,edit
      mask CallbackString:
      | % fft_size = eval(get_param(gcb, 'FFTSize'));
      | % old_vec = eval(get_param(gcb, 'mult_spec'));
      | 
      | % vec = 2.*ones(1,fft_size);
      | % old_size = length(old_vec);
      | 
      | % if(old_size <= fft_size),
      | %    size = old_size;
      | % else,
      | %     size = fft_size;
      | % end
      | 
      | % for n = 1:size, vec(n) = old_vec(n); end
      | % set_param(gcb, 'mult_spec', mat2str(vec));|||||||||||||specify_mult = get_param(gcb,'specify_mult');
      | visibs = get_param(gcb, 'MaskVisibilities');
      | enables = get_param(gcb, 'MaskEnables');
      | enables{15} = 'on';
      | if( strcmp(specify_mult,'off')), visibs{15} = 'off';
      | else, visibs{15} = 'on';
      | end
      | set_param(gcb, 'MaskEnables', enables);
      | set_param(gcb, 'MaskVisibilities', visibs);
      | |% vec = eval( get_param(gcb, 'mult_spec'));
      | % vec_size = length(vec);
      | % fft_size = eval( get_param(gcb, 'FFTSize'));
      | % new_vec = 2.*ones(1, fft_size);
      | 
      | % if(vec_size <= fft_size), size = vec_size;
      | % else size = fft_size;
      | % end
      | 
      | % for n=1:size
      | %     new_vec(n) = vec(n);
      | % end
      | % set_param(gcb, 'mult_spec', mat2str(new_vec));
  pfb_fir_real : Subsystem  AncestorBlock=casper_library/PFBs/pfb_fir_real  mask(pfb_fir_real){PFBSize=11, TotalTaps=4, WindowType=hamming, n_inputs=2, MakeBiplex=0, BitWidthIn=8, BitWidthOut=25, CoeffBitWidth=18, CoeffDistMem=0, add_latency=3, mult_latency=3, bram_latency=2, quantization=Truncate, fwidth=1, specify_mult=off, mult_spec=[0 1 2 0]}
      mask prompts: PFBSize "Size of PFB: (2^? pnts)"; TotalTaps "Total Number of Taps:"; WindowType "Windowing Function:"; n_inputs "Number of Simultaneous Inputs: (2^?)"; MakeBiplex "Make Biplex"; BitWidthIn "Input Bitwidth:"; BitWidthOut "Output Bitwidth:"; CoeffBitWidth "Coefficient Bitwidth:"; CoeffDistMem "Use Distributed Memory for Coeffs"; add_latency "Add Latency"; mult_latency "Mult Latency"; bram_latency "BRAM Latency"; quantization "Quantization Behavior"; fwidth "Bin Width Scaling (normal=1)"; specify_mult "Specify multiplier use (embedded if not specified)"; mult_spec "Multiplier specification (0=core, 1=embedded, 2=behavioural) (left=1st tap)"
      mask init:
      | pfb_fir_real_init(gcb,...
      |     'PFBSize', PFBSize,...
      |     'TotalTaps', TotalTaps,...
      |     'WindowType', WindowType,...
      |     'n_inputs', n_inputs,...
      |     'MakeBiplex', MakeBiplex,...
      |     'BitWidthIn', BitWidthIn,...
      |     'BitWidthOut', BitWidthOut,...
      |     'CoeffBitWidth', CoeffBitWidth,...
      |     'CoeffDistMem', CoeffDistMem,...
      |     'add_latency', add_latency,...
      |     'mult_latency', mult_latency,...
      |     'bram_latency', bram_latency,...
      |     'quantization', quantization,...
      |     'fwidth', fwidth,...
      |     'specify_mult', specify_mult,...
      |     'mult_spec', mult_spec);
      settings: AttributesFormatString=taps=4, add_latency=3
      mask Help: eval('xlWeb([getenv(''MLIB_ROOT''), ''\doc\htmlblocks\sp_pfb_fir_real\sp_pfb_fir_real.html''])')
      mask StyleString: edit,edit,popup(bartlett|barthannwin|blackman|blackmanharris|bohamwin|chebwin|flattopwin|gausswin|hamming|hann|kaiser|nuttallwin|parzenwin|rectwin|tukeywin|triang|userwindow),edit,edit,edit,edit,edit,edit,edit,edit,edit,popup(Truncate|Round  (unbiased: +/- Inf)|Round  (unbiased: Even Values)),edit,checkbox,edit
      mask CallbackString:
      | |num_taps = eval(get_param(gcb, 'TotalTaps'));
      | old_vec = eval(get_param(gcb, 'mult_spec'));
      | 
      | vec = ones(1,num_taps);
      | old_size = length(old_vec);
      | 
      | if(old_size <= num_taps),
      |     size = old_size;
      | else,
      |     size = num_taps;
      | end
      | 
      | for n = 1:size, vec(n) = old_vec(n); end
      | set_param(gcb, 'mult_spec', mat2str(vec));|||||||||||||specify_mult = get_param(gcb,'specify_mult');
      | if( strcmp(specify_mult,'off')),
      |     set_param(gcb, 'MaskEnables', {'on','on','on','on','on','on','on','on','on','on','on','on','on','on','on','off'});
      | else
      |     set_param(gcb, 'MaskEnables', {'on','on','on','on','on','on','on','on','on','on','on','on','on','on','on','on'});
      | end
      | 
      | |vec = eval( get_param(gcb, 'mult_spec'));
      | vec_size = length(vec);
      | num_taps = eval( get_param(gcb, 'TotalTaps'));
      | new_vec = ones(1, num_taps);
      | 
      | if(vec_size <= num_taps), size = vec_size;
      | else size = num_taps;
      | end
      | 
      | for n=1:size
      |     new_vec(n) = vec(n);
      | end
      | set_param(gcb, 'mult_spec', mat2str(new_vec));
  sync_o : Outport
  out0 : Outport  Port=2
  out1 : Outport  Port=3
  of : Outport  Port=4
  wires:
  pfb_fir_real/1(sync_out) -> Delay1/1
  Constant1/1 -> fft_wideband_real1/2(shift)
  Delay1/1 -> fft_wideband_real1/1(sync)
  pfb_fir_real/2(pol1_out1) -> Shift7/1
  pfb_fir_real/3(pol1_out2) -> Shift6/1
  pfb_fir_real/4(pol1_out3) -> Shift5/1
  pfb_fir_real/5(pol1_out4) -> Shift4/1
  Shift7/1 -> fft_wideband_real1/3(in0)
  Shift6/1 -> fft_wideband_real1/4(in1)
  Shift5/1 -> fft_wideband_real1/5(in2)
  Shift4/1 -> fft_wideband_real1/6(in3)
  sync/1 -> pfb_fir_real/1(sync)
  in0/1 -> pfb_fir_real/2(pol1_in1)
  in1/1 -> pfb_fir_real/3(pol1_in2)
  in2/1 -> pfb_fir_real/4(pol1_in3)
  in3/1 -> pfb_fir_real/5(pol1_in4)
  fft_wideband_real1/1(sync_out) -> sync_o/1
  fft_wideband_real1/2(out0) -> out0/1
  fft_wideband_real1/3(out1) -> out1/1
  fft_wideband_real1/4(of) -> of/1

== system rmspec/pol_reorder ==
  sync : Inport
  In1 : Inport  Port=2
  In2 : Inport  Port=3
  Concat : xbsIndex_r4/Concat  num_inputs=2  dbl_ovrd=off  block_type=concat
      settings: block_version=10.1.3
  Concat1 : xbsIndex_r4/Concat  num_inputs=2  dbl_ovrd=off  block_type=concat
      settings: block_version=10.1.3
  Constant5 : xbsIndex_r4/Constant  arith_type=Boolean  const=1  n_bits=1  bin_pt=0  explicit_period=on  period=1  equ=P=C  opselect=C  inp2=PCIN>>17  opr=+  inp1=P  carry=CIN  dbl_ovrd=off  block_type=constant
  Delay{1..2,16..17} (4 alike) : xbsIndex_r4/Delay  en=off  latency=1  dbl_ovrd=off  reg_retiming=off  block_type=delay
  Mux : xbsIndex_r4/Mux  inputs=2  en=off  latency=0  precision=Full  arith_type=Unsigned  n_bits=16  bin_pt=14  quantization=Truncate  overflow=Wrap  dbl_ovrd=off  block_type=mux
  Slice : xbsIndex_r4/Slice  nbits=18  boolean_output=off  mode=Lower Bit Location + Width  bit1=0  base1=LSB of Input  bit0=18  base0=LSB of Input  dbl_ovrd=off  block_type=slice
      settings: infoedit="Extracts a given range of bits from each input sample and presents it at the output.  The output type is ordinarily unsigned with binary point at zero, but can be Boolean when the slice is one bit wide.<P><P>Hardware notes: In hardware this block costs nothing."  block_version=10.1.3
  Slice1 : xbsIndex_r4/Slice  nbits=18  boolean_output=off  mode=Lower Bit Location + Width  bit1=0  base1=LSB of Input  bit0=0  base0=LSB of Input  dbl_ovrd=off  block_type=slice
      settings: infoedit="Extracts a given range of bits from each input sample and presents it at the output.  The output type is ordinarily unsigned with binary point at zero, but can be Boolean when the slice is one bit wide.<P><P>Hardware notes: In hardware this block costs nothing."  block_version=10.1.3
  Terminator5 : Terminator
  reorder : Subsystem  AncestorBlock=casper_library/Reorder/reorder  mask(reorder){map=getfield( getfield( get_param( gcb,'UserData' ), 'parameters'),'map'), n_inputs=1, bram_latency=3, map_latency=3, double_buffer=0}
      mask prompts: map "Output Order:"; n_inputs "Number of inputs"; bram_latency "BRAM Latency"; map_latency "Map Latency"; double_buffer "Double Buffer"
      mask init:
      | reorder_init(gcb, ...
      |     'map', map, ...
      |     'n_inputs', n_inputs, ...
      |     'bram_latency', bram_latency, ...
      |     'map_latency', map_latency, ...
      |     'double_buffer', double_buffer);
      settings: AttributesFormatString=order=10
      mask Help: eval('xlWeb([getenv(''MLIB_ROOT''), ''\doc\htmlblocks\sp_reorder\sp_reorder.html''])')
  toggler : xbsIndex_r4/Counter  cnt_type=Free Running  cnt_to=Inf  operation=Up  start_count=0  cnt_by_val=1  arith_type=Unsigned  n_bits=1  bin_pt=0  load_pin=off  rst=on  en=off  explicit_period=on  period=1  dbl_ovrd=off  use_behavioral_HDL=off  use_rpm=off  implementation=Fabric  block_type=counter
  sync_o : Outport
  Out1 : Outport  Port=2
  Out2 : Outport  Port=3
  wires:
  toggler/1 -> Mux/1
  sync/1 -> Delay1/1
  In1/1 -> Delay16/1, Concat/2
  In2/1 -> Delay17/1
  Delay1/1 -> toggler/1, reorder/1(sync)
  Delay16/1 -> Concat/1
  Delay17/1 -> Delay2/1, Concat1/2
  Delay2/1 -> Concat1/1
  Concat1/1 -> Mux/3
  Concat/1 -> Mux/2
  Slice/1 -> Out1/1
  Slice1/1 -> Out2/1
  Constant5/1 -> reorder/2(en)
  Mux/1 -> reorder/3(din0)
  reorder/1(sync_out) -> sync_o/1
  reorder/2(valid) -> Terminator5/1
  reorder/3(dout0) -> Slice/1, Slice1/1

== system rmspec/power_det ==
  sync : Inport
  i0 : Inport  Port=2
  i1 : Inport  Port=3
  Delay1 : xbsIndex_r4/Delay  en=off  latency=1  dbl_ovrd=off  reg_retiming=off  block_type=delay
  Delay2 : xbsIndex_r4/Delay  en=off  latency=6  dbl_ovrd=off  reg_retiming=off  block_type=delay
  Delay3 : xbsIndex_r4/Delay  en=off  latency=1  dbl_ovrd=off  reg_retiming=off  block_type=delay
  Delay4 : xbsIndex_r4/Delay  en=off  latency=1  dbl_ovrd=off  reg_retiming=off  block_type=delay
  Reinterpret1 : xbsIndex_r4/Reinterpret  force_arith_type=on  arith_type=Unsigned  force_bin_pt=on  bin_pt=0  block_type=reinterpret
      settings: infoedit="Changes signal type without altering the binary representation.   You can changed the signal between signed and unsigned, and relocate the binary point.<P><P>Hardware notes: In hardware this block costs nothing.<P><P>Example:  Suppose the input is 6 bits wide, signed, with 2 fractional bits, and the output is forced to unsigned with 0 fractional bits.  Then an input of -2.0 (1110.00 in binary 2's complement) becomes an output of 56 (111000 in binary)."  block_version=10.1.3
  Reinterpret6 : xbsIndex_r4/Reinterpret  force_arith_type=on  arith_type=Unsigned  force_bin_pt=on  bin_pt=0  block_type=reinterpret
      settings: infoedit="Changes signal type without altering the binary representation.   You can changed the signal between signed and unsigned, and relocate the binary point.<P><P>Hardware notes: In hardware this block costs nothing.<P><P>Example:  Suppose the input is 6 bits wide, signed, with 2 fractional bits, and the output is forced to unsigned with 0 fractional bits.  Then an input of -2.0 (1110.00 in binary 2's complement) becomes an output of 56 (111000 in binary)."  block_version=10.1.3
  Slice : xbsIndex_r4/Slice  nbits=18  boolean_output=off  mode=Upper Bit Location + Width  bit1=0  base1=MSB of Input  bit0=7  base0=LSB of Input  dbl_ovrd=off  block_type=slice
      settings: infoedit="Extracts a given range of bits from each input sample and presents it at the output.  The output type is ordinarily unsigned with binary point at zero, but can be Boolean when the slice is one bit wide.<P><P>Hardware notes: In hardware this block costs nothing."  block_version=10.1.3
  Slice1 : xbsIndex_r4/Slice  nbits=18  boolean_output=off  mode=Upper Bit Location + Width  bit1=0  base1=MSB of Input  bit0=7  base0=LSB of Input  dbl_ovrd=off  block_type=slice
      settings: infoedit="Extracts a given range of bits from each input sample and presents it at the output.  The output type is ordinarily unsigned with binary point at zero, but can be Boolean when the slice is one bit wide.<P><P>Hardware notes: In hardware this block costs nothing."  block_version=10.1.3
  power0 : Subsystem  mask(power){BitWidth=18, add_latency=3, mult_latency=3}
      mask prompts: BitWidth "Bit Width"; add_latency "Add Latency"; mult_latency "Mult Latency"
      mask help: Squares real and imaginary components of complex input and adds them.
      mask Help: eval('xlWeb([getenv(''MLIB_ROOT''), ''\doc\htmlblocks\sp_power\sp_power.html''])')
      mask Display:
      | port_label('input', 1, 'c');
      | port_label('output', 1, 'power');
      | disp(['Z^-', num2str(mult_latency+add_latency)]);
  power1 : Subsystem  mask(power){BitWidth=18, add_latency=3, mult_latency=3}
      mask prompts: BitWidth "Bit Width"; add_latency "Add Latency"; mult_latency "Mult Latency"
      mask help: Squares real and imaginary components of complex input and adds them.
      mask Help: eval('xlWeb([getenv(''MLIB_ROOT''), ''\doc\htmlblocks\sp_power\sp_power.html''])')
      mask Display:
      | port_label('input', 1, 'c');
      | port_label('output', 1, 'power');
      | disp(['Z^-', num2str(mult_latency+add_latency)]);
  synco : Outport
  p0 : Outport  Port=2
  p1 : Outport  Port=3
  wires:
  Delay2/1 -> Delay1/1
  sync/1 -> Delay2/1
  power1/1(power) -> Reinterpret1/1
  i1/1 -> power1/1(c)
  power0/1(power) -> Reinterpret6/1
  i0/1 -> power0/1(c)
  Reinterpret6/1 -> Slice/1
  Reinterpret1/1 -> Slice1/1
  Slice/1 -> Delay4/1
  Slice1/1 -> Delay3/1
  Delay1/1 -> synco/1
  Delay3/1 -> p1/1
  Delay4/1 -> p0/1
